simulink model "TimeScaleTEST_sim"  (Simulink 7.8)
settings: Solver=ode8  StartTime=0.0  StopTime=10.0  FixedStep=0.1  RelTol=1e-3
settings Model: Creator=Administrator  LastModifiedBy=Administrator

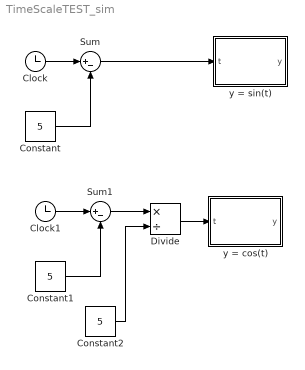
== system TimeScaleTEST_sim ==
  Clock : Clock
  Clock1 : Clock
  Constant : Constant  Value=5
  Constant1 : Constant  Value=5
  Constant2 : Constant  Value=5
  Divide : Product  Inputs=*/
  Sum : Sum  Inputs=|+-
  Sum1 : Sum  Inputs=|+-
  y = cos(t) : MATLAB Function  TreatAsAtomicUnit=on
  y = sin(t) : MATLAB Function  TreatAsAtomicUnit=on
  wires:
  Clock/1 -> Sum/1
  Constant/1 -> Sum/2
  Sum/1 -> y = sin(t)/1(t)
  Clock1/1 -> Sum1/1
  Constant1/1 -> Sum1/2
  Sum1/1 -> Divide/1
  Constant2/1 -> Divide/2
  Divide/1 -> y = cos(t)/1(t)

== matlab function y = cos(t) ==
  data: t input double; y output double
function y = fcn(t)
%#codegen

y = cos(t);
end

== matlab function y = sin(t) ==
  data: t input double; y output double
function y = fcn(t)
%#codegen

y = sin(t);
end
